simulink library "oneTetherThreeSurfaceCtrl_cl"  (R2018b)
settings: Solver=VariableStepAuto  StartTime=0.0  StopTime=10.0  RelTol=1e-3
undefined symbols (not defined in the file or in its folder): ctrl, initializeBussesFromBlock
libraries: filteredPIDController_ul x3
settings Model: Creator=mcobb  LastModifiedBy=mcobb

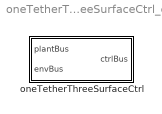
== system oneTetherThreeSurfaceCtrl_cl ==
  oneTetherThreeSurfaceCtrl : Subsystem  LoadFcn=initializeBussesFromBlock(gcb)  InitFcn=initializeBussesFromBlock(gcb)  StartFcn=initializeBussesFromBlock(gcb)  VariantControl=VSS_controller_oneTetherThreeSurfaceCtrl

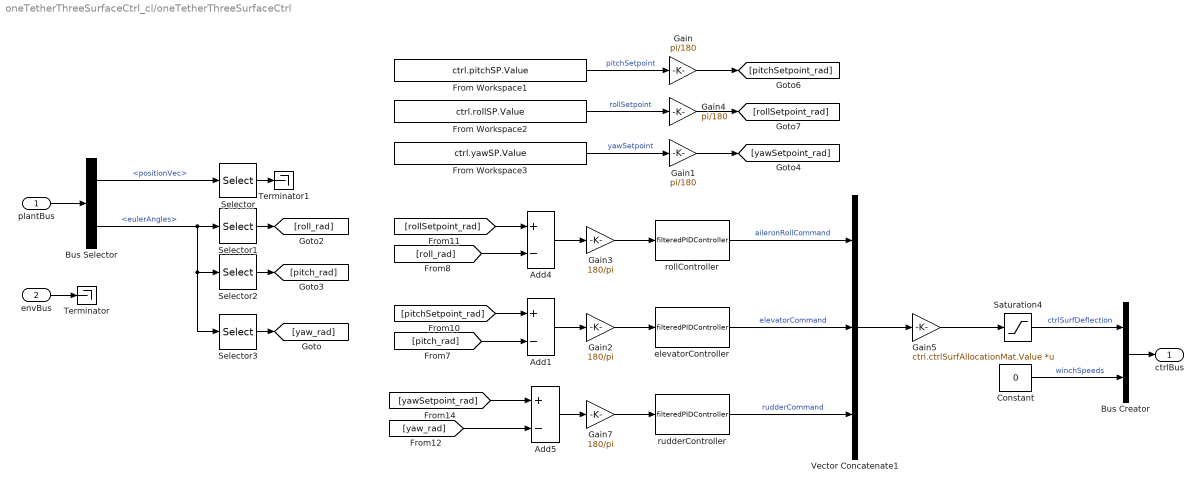
== system oneTetherThreeSurfaceCtrl_cl/oneTetherThreeSurfaceCtrl ==
  plantBus : Inport  OutDataTypeStr=Bus: plantBus
  envBus : Inport  Port=2  OutDataTypeStr=Bus: envBus
  Add1 : Sum  Inputs=+-
  Add4 : Sum  Inputs=+-
  Add5 : Sum  Inputs=+-
  Bus Creator : BusCreator  Inputs=2  OutDataTypeStr=Bus: fltCtrlBus
  Bus Selector : BusSelector  OutputSignals=positionVec,eulerAngles
  Constant : Constant  Value=0
  From Workspace1 : FromWorkspace  VariableName=ctrl.pitchSP.Value  SampleTime=0
  From Workspace2 : FromWorkspace  VariableName=ctrl.rollSP.Value  SampleTime=0
  From Workspace3 : FromWorkspace  VariableName=ctrl.yawSP.Value  SampleTime=0
  Gain : Gain  Gain=pi/180
  Gain1 : Gain  Gain=pi/180
  Gain2 : Gain  Gain=180/pi
  Gain3 : Gain  Gain=180/pi
  Gain4 : Gain  Gain=pi/180
  Gain5 : Gain  Gain=ctrl.ctrlSurfAllocationMat.Value  Multiplication=Matrix(K*u)
  Gain7 : Gain  Gain=180/pi
  Saturation4 : Saturate  UpperLimit=ctrl.outputSat.upperLimit.Value  LowerLimit=ctrl.outputSat.lowerLimit.Value
  Selector : Selector  InputPortWidth=3  IndexOptions=Index vector (dialog)  Indices=3  OutputSizes=1
  Selector1 : Selector  InputPortWidth=3  IndexOptions=Index vector (dialog)  Indices=1  OutputSizes=1
  Selector2 : Selector  InputPortWidth=3  IndexOptions=Index vector (dialog)  Indices=2  OutputSizes=1
  Selector3 : Selector  InputPortWidth=3  IndexOptions=Index vector (dialog)  Indices=3  OutputSizes=1
  Terminator : Terminator
  Terminator1 : Terminator
  Vector Concatenate1 : Concatenate  NumInputs=3
  elevatorController : filteredPIDController_ul/filteredPIDController  kp=ctrl.elevators.kp.Value  ki=ctrl.elevators.ki.Value  kd=ctrl.elevators.kd.Value  Value=ctrl.elevators.tau.Value
  rollController : filteredPIDController_ul/filteredPIDController  kp=ctrl.ailerons.kp.Value  ki=ctrl.ailerons.ki.Value  kd=ctrl.ailerons.kd.Value  Value=ctrl.ailerons.tau.Value
  rudderController : filteredPIDController_ul/filteredPIDController  kp=ctrl.rudder.kp.Value  ki=ctrl.rudder.ki.Value  kd=ctrl.rudder.kd.Value  Value=ctrl.rudder.tau.Value
  ctrlBus : Outport  OutDataTypeStr=Bus: fltCtrlBus
  wires:
  Saturation4/1 -> Bus Creator/1  "ctrlSurfDeflection"
  elevatorController/1 -> Vector Concatenate1/2  "elevatorCommand"
  [pitch_rad] -> Add1/2
  Vector Concatenate1/1 -> Gain5/1
  Gain2/1 -> elevatorController/1
  Add1/1 -> Gain2/1
  Bus Creator/1 -> ctrlBus/1
  Constant/1 -> Bus Creator/2  "winchSpeeds"
  envBus/1 -> Terminator/1
  plantBus/1 -> Bus Selector/1
  Gain/1 -> [pitchSetpoint_rad]
  Gain4/1 -> [rollSetpoint_rad]
  Selector/1 -> Terminator1/1
  [pitchSetpoint_rad] -> Add1/1
  Bus Selector/1 -> Selector/1  "<positionVec>"
  Bus Selector/2 -> Selector3/1, Selector2/1, Selector1/1  "<eulerAngles>"
  Selector1/1 -> [roll_rad]
  Selector2/1 -> [pitch_rad]
  From Workspace1/1 -> Gain/1  "pitchSetpoint"
  From Workspace2/1 -> Gain4/1  "rollSetpoint"
  [yawSetpoint_rad] -> Add5/1
  Add5/1 -> Gain7/1
  rudderController/1 -> Vector Concatenate1/3  "rudderCommand"
  Gain7/1 -> rudderController/1
  [yaw_rad] -> Add5/2
  From Workspace3/1 -> Gain1/1  "yawSetpoint"
  Gain1/1 -> [yawSetpoint_rad]
  Selector3/1 -> [yaw_rad]
  Gain5/1 -> Saturation4/1
  Gain3/1 -> rollController/1
  Add4/1 -> Gain3/1
  [roll_rad] -> Add4/2
  [rollSetpoint_rad] -> Add4/1
  rollController/1 -> Vector Concatenate1/1  "aileronRollCommand"
